simulink model "Khaldoun_Multivariable"  (Simulink 7.9)
settings: Solver=ode45  StartTime=0.0  StopTime=1.5  RelTol=1e-3
InitFcn:
  | k = 1.381e-23;
  | q = 1.602e-19;
  | A = 1.81;
  | Eg = 1.16;
  | Ns = 72;
  | Np=1;
  | ki=1.96e-3;
  | Rs =2.48e-3;
  | Rp = 8.7;
  | Tr =298.5;
  | I0_r = 1.13e-6;
  | Ir_ph = 5.61;
  | 
  | T=298.5;
  | 
  | Ts_Power=5e-6;
  | Ts=5e-6;
  | Ts_Control=10e-6;
  | 
  | Ci=100;
  | C1i=42;
  | D0=0.5;
  | 
  | C=440e-6;
  | L=440e-6;
  | C1=22e-6;
  | 
  | sol=1;
  | 
  | C_init=100;
  | C1_init=42;
  | L1_init=5;
  | 
  | 
  | kg=0.005;
  | a=0.02;
  | wl=50;
  | wh=45;
  | 
  | w1=4500;
  | w2=6500;
  | w3=8500;
  | w4=5500;
  | w5=7500;
  | w6=9500;
StartFcn:
  | k = 1.381e-23;
  | q = 1.602e-19;
  | A = 1.81;
  | Eg = 1.16;
  | Ns = 72;
  | Np=1;
  | ki=1.96e-3;
  | Rs =2.48e-3;
  | Rp = 8.7;
  | Tr =298.5;
  | I0_r = 1.13e-6;
  | Ir_ph = 5.61;
  | 
  | T=298.5;
  | 
  | Ts_Power=5e-6;
  | Ts=5e-6;
  | Ts_Control=10e-6;
  | 
  | Ci=100;
  | C1i=42;
  | D0=0.5;
  | 
  | C=440e-6;
  | L=440e-6;
  | C1=22e-6;
  | 
  | sol=1;
  | 
  | C_init=100;
  | C1_init=42;
  | L1_init=5;
  | 
  | 
  | 
  | kg=0.005;
  | a=0.02;
  | wl=50;
  | wh=45;
  | 
  | w1=4500;
  | w2=6500;
  | w3=8500;
  | w4=5500;
  | w5=7500;
  | w6=9500;
undefined symbols (not defined in the file or in its folder): D1, Delta, sigbuilder_block
libraries: powerlib x99, powerlib_extras x3, simulink x2
(part 1 of 2)
settings Model: Creator=Khaled  LastModifiedBy=Khaled

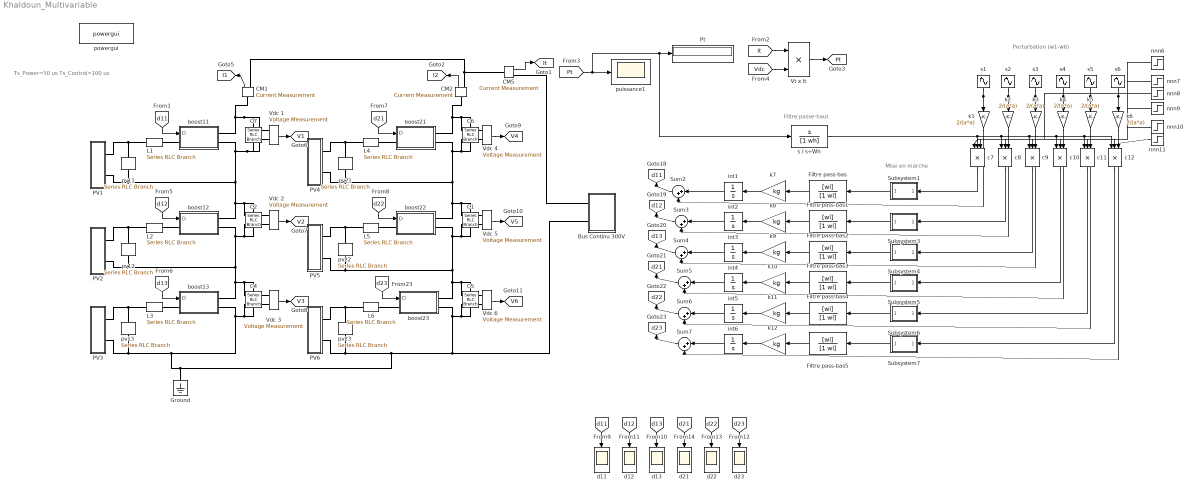
== system Khaldoun_Multivariable ==
  note: Ts_Power=50 us
      | Ts_Control=100 us
  note: Filtre passe-haut
  note: Mise en marche
  note: Perturbation (w1-w6)
  Bus Continu 300V : Subsystem
  C{1..2,4..7} (6 alike) : powerlib/Elements/Series RLC Branch  LConnTagsString=__new0  RConnTagsString=__new0  BranchType=C  Resistance=1.0  Inductance=1.0  SetiL0=off  InitialCurrent=0  Capacitance=C  Setx0=on  InitialVoltage=Ci  Measurements=None
  CM1 : powerlib/Measurements/Current Measurement  Tag=PoWeRsYsTeMmEaSuReMeNt  PhasorSimulation=off  OutputType=Magnitude  PSBequivalent=0
  CM2 : powerlib/Measurements/Current Measurement  Tag=PoWeRsYsTeMmEaSuReMeNt  PhasorSimulation=off  OutputType=Magnitude  PSBequivalent=0
  CM5 : powerlib/Measurements/Current Measurement  Tag=PoWeRsYsTeMmEaSuReMeNt  PhasorSimulation=off  OutputType=Magnitude  PSBequivalent=0
  Filtre pass-bas{,1..5} (6 alike) : TransferFcn  Numerator=[wl]  Denominator=[1 wl]
  Ground : powerlib/Elements/Ground  LConnTagsString=a
  L{1..6} (6 alike) : powerlib/Elements/Series RLC Branch  LConnTagsString=__new0  RConnTagsString=__new0  BranchType=L  Resistance=1.0  Inductance=L  SetiL0=on  InitialCurrent=L1_init  Capacitance=1.0  Setx0=off  InitialVoltage=0  Measurements=None
  PV1 : Subsystem  RequirementInfo={} %GIDa_ec48a4a5_e8ed_46b8_b352_e7f6805c7ac6
  PV2 : Subsystem  RequirementInfo={} %GIDa_9735ab26_5599_4b61_891e_3252a34807da
  PV3 : Subsystem  RequirementInfo={} %GIDa_8edbe910_4089_49ae_850f_62c7b8a72111
  PV4 : Subsystem  RequirementInfo={} %GIDa_f6f8a1f9_a3e9_414c_b28d_369a8e09ef45
  PV5 : Subsystem  RequirementInfo={} %GIDa_1a594654_d930_4a6d_9a1b_d857bde8c8a5
  PV6 : Subsystem  RequirementInfo={} %GIDa_cee78ba7_daff_4548_90a5_e4e442d265c0
  Pt : Display
      settings: Format=bank  Decimation=100
  Subsystem1 : Subsystem
  Subsystem3 : Subsystem
  Subsystem4 : Subsystem
  Subsystem5 : Subsystem
  Subsystem6 : Subsystem
  Subsystem7 : Subsystem
  Sum{2..7} (6 alike) : Sum  Inputs=|++
  Vdc {1..6} (6 alike) : powerlib/Measurements/Voltage Measurement  Tag=PoWeRsYsTeMmEaSuReMeNt  PhasorSimulation=off  OutputType=Magnitude  PSBequivalent=0
  Vt x It : Product  RndMeth=Zero
  boost11 : Subsystem
  boost12 : Subsystem
  boost13 : Subsystem
  boost21 : Subsystem
  boost22 : Subsystem
  boost23 : Subsystem
  c{7..12} (6 alike) : Product  Inputs=3  RndMeth=Zero
  d{11..13,21..23} (6 alike) : Scope
      d11 settings: TimeRange=1  YMin=582  YMax=599  SaveName=mv6  Decimation=100
      d12 settings: TimeRange=1  YMin=582  YMax=599  SaveName=mv1  Decimation=100
      d13 settings: TimeRange=1  YMin=582  YMax=599  SaveName=mv2  Decimation=100
      d21 settings: TimeRange=1  YMin=582  YMax=599  SaveName=mv3  Decimation=100
      d22 settings: TimeRange=1  YMin=582  YMax=599  SaveName=mv4  Decimation=100
      d23 settings: TimeRange=1  YMin=582  YMax=599  SaveName=mv5  Decimation=100
  int{1..6} (6 alike) : Integrator  InitialCondition=0.5  LimitOutput=on  UpperSaturationLimit=0.8  LowerSaturationLimit=0.2
  k{1..6} (6 alike) : Gain  Gain=2/(a*a)
  k{7..12} (6 alike) : Gain  Gain=kg
  nnn{6..11} (6 alike) : Step  Time=0.2  SampleTime=0
  powergui : powerlib/powergui  Priority=1  SimulationMode=Discrete  SolverType=Tustin  SampleTime=Ts_Power  frequency=60  SPID=off  DisableSnubberDevices=off  DisableRonSwitches=off  DisableVfSwitches=off  SwTol=0  Interpol=off  DisplayEquations=off  FunctionMessages=off  frequencyindice=0  Pbase=100e6  ErrMax=1e-4  Iterations=50  UnitsV=kV  UnitsW=MW  echomessages=off  HookPort=off  EnableUseOfTLC=off  x0status=blocks  RestoreLinks=warning  ResistiveCurrentMeasurement=off  Frange=[0:2:500]  Ylog=off  Xlog=on  ShowGrid=off  save=off  variable=ZData  ZoomFFT=on  StartTime=0.0  cycles=1  DisplayStyle=1  fundamental=60  FreqAxis=off  MaxFrequency=1000  frequencyindicesteady=1  RmsSteady=1  display=off  Ts=0  methode=off
  puissance1 : Scope
      settings: TimeRange=1  YMin=0  YMax=1400  SaveName=mv  Decimation=100
  pv{11..13,21..23} (6 alike) : powerlib/Elements/Series RLC Branch  LConnTagsString=__new0  RConnTagsString=__new0  BranchType=C  Resistance=0.01  Inductance=1.0  SetiL0=off  InitialCurrent=0  Capacitance=C1  Setx0=on  InitialVoltage=C1_init  Measurements=None
  s / s+Wh : TransferFcn  Numerator=[1 0]  Denominator=[1 wh]  AbsoluteTolerance=1e-6
  s1 : Sin  Amplitude=a  Frequency=w1/(2*pi)  SampleTime=0
  s2 : Sin  Amplitude=a  Frequency=w2/(2*pi)  SampleTime=0
  s3 : Sin  Amplitude=a  Frequency=w3/(2*pi)  SampleTime=0
  s4 : Sin  Amplitude=a  Frequency=w4/(2*pi)  SampleTime=0
  s5 : Sin  Amplitude=a  Frequency=w5/(2*pi)  SampleTime=0
  s6 : Sin  Amplitude=a  Frequency=w6/(2*pi)  SampleTime=0
  tag scope: I1=global, I2=global, It=global, Pt=global, V1=global, V2=global, V3=global, V4=global, V5=global, V6=global, d11=global, d12=global, d13=global, d21=global, d22=global, d23=global
  wires:
  [It] -> Vt x It/1
  Vt x It/1 -> [Pt]
  [Vdc] -> Vt x It/2
  [Pt] -> puissance1/1, Pt/1, s / s+Wh/1
  s1/1 -> k1/1, Sum2/2
  s2/1 -> k2/1, Sum3/2
  s3/1 -> k3/1, Sum4/2
  s4/1 -> k4/1, Sum5/2
  s5/1 -> k5/1, Sum6/2
  s6/1 -> k6/1, Sum7/2
  k1/1 -> c7/2
  k2/1 -> c8/2
  k3/1 -> c9/2
  k4/1 -> c10/2
  k5/1 -> c11/2
  k6/1 -> c12/2
  c7/1 -> Subsystem1/1(In1)
  c8/1 -> Subsystem3/1(In1)
  c9/1 -> Subsystem4/1(In1)
  c10/1 -> Subsystem5/1(In1)
  c11/1 -> Subsystem6/1(In1)
  c12/1 -> Subsystem7/1(In1)
  Filtre pass-bas/1 -> k7/1
  Filtre pass-bas1/1 -> k8/1
  Filtre pass-bas2/1 -> k9/1
  Filtre pass-bas3/1 -> k10/1
  Filtre pass-bas4/1 -> k11/1
  Filtre pass-bas5/1 -> k12/1
  k7/1 -> int1/1
  k8/1 -> int2/1
  k9/1 -> int3/1
  k10/1 -> int4/1
  k11/1 -> int5/1
  k12/1 -> int6/1
  int1/1 -> Sum2/1
  int2/1 -> Sum3/1
  int3/1 -> Sum4/1
  int4/1 -> Sum5/1
  int5/1 -> Sum6/1
  int6/1 -> Sum7/1
  Sum2/1 -> [d11]
  Sum3/1 -> [d12]
  Sum4/1 -> [d13]
  Sum5/1 -> [d21]
  Sum6/1 -> [d22]
  Sum7/1 -> [d23]
  nnn6/1 -> c7/3
  nnn7/1 -> c8/3
  nnn8/1 -> c9/3
  nnn9/1 -> c10/3
  nnn10/1 -> c11/3
  nnn11/1 -> c12/3
  Subsystem1/1(Out1) -> Filtre pass-bas/1
  Subsystem3/1(Out1) -> Filtre pass-bas1/1
  Subsystem4/1(Out1) -> Filtre pass-bas2/1
  Subsystem5/1(Out1) -> Filtre pass-bas3/1
  Subsystem6/1(Out1) -> Filtre pass-bas4/1
  Subsystem7/1(Out1) -> Filtre pass-bas5/1
  s / s+Wh/1 -> c7/1, c8/1, c9/1, c10/1, c11/1, c12/1
  CM5/1 -> [It]
  CM1/1 -> [I1]
  CM2/1 -> [I2]
  Vdc 1/1 -> [V1]
  Vdc 2/1 -> [V2]
  Vdc 3/1 -> [V3]
  Vdc 6/1 -> [V6]
  Vdc 5/1 -> [V5]
  Vdc 4/1 -> [V4]
  [d11] -> d11/1
  [d12] -> d12/1
  [d13] -> d13/1
  [d21] -> d21/1
  [d22] -> d22/1
  [d23] -> d23/1
  [d11] -> boost11/1(D)
  [d12] -> boost12/1(D)
  [d13] -> boost13/1(D)
  [d21] -> boost21/1(D)
  [d22] -> boost22/1(D)
  [d23] -> boost23/1(D)
  connections:
  PV2/RConn1 -- pv12/LConn1 -- L2/RConn1
  PV3/RConn1 -- L3/RConn1 -- pv13/LConn1
  pv11/RConn1 -- PV1/RConn2 -- boost11/RConn2 -- Vdc 1/LConn2 -- C7/RConn1 -- boost12/RConn1 -- Vdc 2/LConn1 -- C2/LConn1
  boost13/RConn1 -- pv12/RConn1 -- PV2/RConn2 -- Vdc 2/LConn2 -- C2/RConn1 -- boost12/RConn2 -- Vdc 3/LConn1 -- C4/LConn1
  PV1/RConn1 -- L1/RConn1 -- pv11/LConn1
  PV5/RConn1 -- pv22/LConn1 -- L5/RConn1
  PV6/RConn1 -- L6/RConn1 -- pv23/LConn1
  boost22/RConn1 -- C6/RConn1 -- Vdc 4/LConn2 -- boost21/RConn2 -- pv21/RConn1 -- PV4/RConn2 -- Vdc 5/LConn1 -- C1/LConn1
  C6/LConn1 -- Vdc 4/LConn1 -- CM2/LConn1 -- boost21/RConn1
  boost23/RConn1 -- pv22/RConn1 -- PV5/RConn2 -- Vdc 5/LConn2 -- C1/RConn1 -- boost22/RConn2 -- Vdc 6/LConn1 -- C5/LConn1
  PV4/RConn1 -- L4/RConn1 -- pv21/LConn1
  CM1/LConn1 -- boost11/RConn1 -- Vdc 1/LConn1 -- C7/LConn1
  CM5/LConn1 -- CM2/RConn1 -- CM1/RConn1
  boost13/RConn2 -- pv13/RConn1 -- PV3/RConn2 -- pv23/RConn1 -- PV6/RConn2 -- Vdc 6/LConn2 -- C5/RConn1 -- boost23/RConn2 -- Bus Continu 300V/LConn2 -- Ground/LConn1 -- Vdc 3/LConn2 -- C4/RConn1
  L3/LConn1 -- boost13/LConn1
  Bus Continu 300V/LConn1 -- CM5/RConn1
  boost21/LConn1 -- L4/LConn1
  L2/LConn1 -- boost12/LConn1
  boost11/LConn1 -- L1/LConn1
  L6/LConn1 -- boost23/LConn1
  L5/LConn1 -- boost22/LConn1

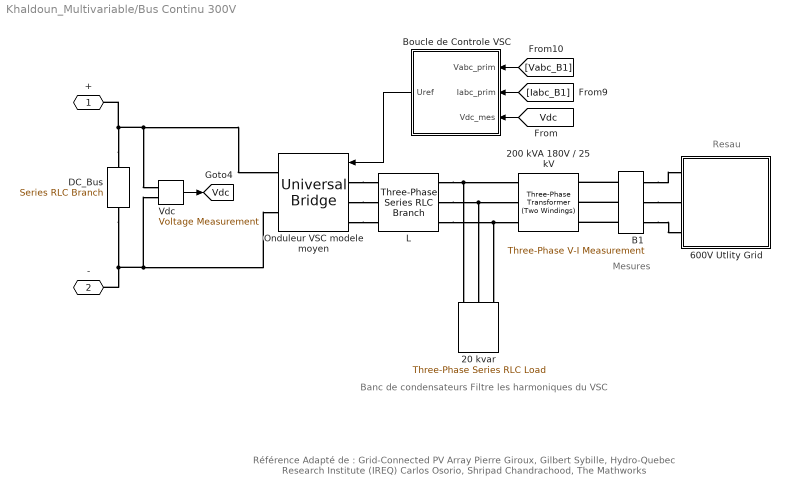
== system Khaldoun_Multivariable/Bus Continu 300V ==
  note: Resau
  note: Banc de condensateurs
      | Filtre les harmoniques du VSC
  note: Mesures
  note: Référence
      | Adapté de :
      | Grid-Connected PV Array
      | Pierre Giroux, Gilbert Sybille, Hydro-Quebec Research Institute (IREQ) Carlos Osorio, Shripad Chandrachood, The Mathworks
  "20 kvar " : powerlib/Elements/Three-Phase Series RLC Load  LConnTagsString=A|B|C  Configuration=Y (grounded)  NominalVoltage=180  NominalFrequency=60  ActivePower=20e3/100  InductivePower=0  CapacitivePower=20e3  Measurements=None  LoadType=constant Z
  200 kVA 180V / 25 kV : powerlib/Elements/Three-Phase Transformer (Two Windings)  Winding1Connection=Yg  UNITS=pu  NominalPower=[200e3 , 60 ]  Winding1=[ 25e3 , 0.001 , 0.03 ]  Winding2Connection=Delta (D1)  Winding2=[ 180 , 0.001 , 0.03 ]  SetSaturation=off  Rm=500  Lm=500  Saturation=[ 0,0 ; 0.0024,1.2 ; 1.0,1.52 ]  Hysteresis=off  DataFile='hysteresis'  SetInitialFlux=off  InitialFluxes=[ 0.8 , -0.8 , 0.7 ]  Measurements=None  MoreParameters=off  BreakLoop=off  DataType=off  TransfoNumber=0
  600V Utlity Grid : Subsystem
  B1 : powerlib/Measurements/Three-Phase V-I Measurement  VoltageMeasurement=phase-to-ground  SetLabelV=on  LabelV=Vabc_B1  Vpu=off  VpuLL=off  CurrentMeasurement=yes  SetLabelI=on  LabelI=Iabc_B1  Ipu=off  Pbase=100e6  Vbase=500e3  OutputType=Magnitude  PhasorSimulation=off  PSBequivalent=0
  Boucle de Controle VSC : Subsystem  mask(VSC Main Controller){nom=[ 200e3  60 ], Vnom=[ 25e3 260 ], Vnom_dc=300, RLxfo=[0.002  0.06 ], RLchoke=[1e-3  125e-6  ], K_VDCreg=[2  800], K_Ireg=[0.3 20], Ts=Ts_Control}
      mask prompts: nom "Puissance et féquence nominales [ Pnom(VA)  Fnom(Hz) ]:"; Vnom "Tension nominale au primaire et secondaire (Vrms LL) [ Vnom_prim   Vnom_sec ]:"; Vnom_dc "Tension du bus DC bus nominale (V):"; RLxfo "Impedance de fuite du transformateur (pu/Pnom) [ Rxfo  Lxf ]"; RLchoke "Impedance choke [ R(ohm) L(H) ]"; K_VDCreg "Gains régulateur de tension du bus DC [ Kp  Ki ]:"; K_Ireg "Gains régulateur du courant du bus D [ Kp  Ki ]:"; Ts "Temps d'échantillonnage"
      mask init:
      | Pnom=nom(1);
      | Fnom=nom(2);
      | Vnom_prim=Vnom(1);
      | Vnom_sec=Vnom(2);
      | Zbase=Vnom_sec^2/Pnom;
      | Rtot_pu=RLxfo(1) + RLchoke(1)/Zbase;
      | Ltot_pu=RLxfo(2) + RLchoke(2)/(Zbase/(2*pi*Fnom));
      | Kp_VDCreg=K_VDCreg(1);
      | Ki_VDCreg=K_VDCreg(2);
      | Kp_Ireg=K_Ireg(1);
      | Ki_Ireg=K_Ireg(2);
      | Vdc_ref=Vnom_dc;
  DC_Bus : powerlib/Elements/Series RLC Branch  LConnTagsString=__new0  RConnTagsString=__new0  BranchType=C  Resistance=1.0  Inductance=1.0  SetiL0=off  InitialCurrent=0  Capacitance=12000e-6  Setx0=on  InitialVoltage=300  Measurements=None
  L : powerlib/Elements/Three-Phase Series RLC Branch  LConnTagsString=A|B|C  RConnTagsString=A|B|C  BranchType=RL  Resistance=0.1  Inductance=125e-6  Capacitance=inf  Measurements=None
  Onduleur VSC modele moyen : powerlib/Power Electronics/Universal Bridge  Arms=3  SnubberResistance=1e5  SnubberCapacitance=inf  Device=Average-model based VSC  Ron=1e-3  Lon=0  ForwardVoltages="[  0  0  ]"  ForwardVoltage=0  GTOparameters=[ 10e-6 , 20e-6 ]  IGBTparameters=[ 1e-6 , 2e-6 ]  Measurements=None  Measurements_2=None  converterType=Rectifier
  "Vdc " : powerlib/Measurements/Voltage Measurement  Tag=PoWeRsYsTeMmEaSuReMeNt  PhasorSimulation=off  OutputType=Magnitude  PSBequivalent=0
  + : PMIOPort  Port=1  Side=Left
  - : PMIOPort  Port=2  Side=Left
  tag scope: Vdc=global
  wires:
  [Vabc_B1] -> Boucle de Controle VSC/1(Vabc_prim)
  [Iabc_B1] -> Boucle de Controle VSC/2(Iabc_prim)
  [Vdc] -> Boucle de Controle VSC/3(Vdc_mes)
  Boucle de Controle VSC/1(Uref) -> Onduleur VSC modele moyen/1
  "Vdc "/1 -> [Vdc]
  connections:
  L/RConn1 -- "20 kvar "/LConn1 -- 200 kVA 180V / 25 kV/RConn1
  L/RConn2 -- "20 kvar "/LConn2 -- 200 kVA 180V / 25 kV/RConn2
  L/RConn3 -- "20 kvar "/LConn3 -- 200 kVA 180V / 25 kV/RConn3
  B1/LConn1 -- 200 kVA 180V / 25 kV/LConn1
  B1/LConn2 -- 200 kVA 180V / 25 kV/LConn2
  B1/LConn3 -- 200 kVA 180V / 25 kV/LConn3
  B1/RConn1 -- 600V Utlity Grid/LConn1
  B1/RConn2 -- 600V Utlity Grid/LConn2
  B1/RConn3 -- 600V Utlity Grid/LConn3
  DC_Bus/LConn1 -- +/RConn1 -- Onduleur VSC modele moyen/RConn1 -- "Vdc "/LConn1
  DC_Bus/RConn1 -- -/RConn1 -- Onduleur VSC modele moyen/RConn2 -- "Vdc "/LConn2
  Onduleur VSC modele moyen/LConn1 -- L/LConn1
  Onduleur VSC modele moyen/LConn2 -- L/LConn2
  Onduleur VSC modele moyen/LConn3 -- L/LConn3

== system Khaldoun_Multivariable/PV1 ==
  Diode : Subsystem
      mask Display:
      | plot(-75,-50,100,150, [-15 -15 43 -15 -15 -75],[50 8 50 92 50 50], ...
      |     [43 43],[8 94],[100 43], [50 50])
  Eclairage : Step  Time=0  Before=1  SampleTime=0
  Iph : powerlib/Electrical Sources/Controlled Current Source  Initialize=on  Source_Type=DC  Amplitude=0  Phase=0  Frequency=0  Measurements=None
  Iph_ : Constant  Value=Ir_ph
  Product1 : Product  Inputs=**  RndMeth=Zero
  Rp : powerlib/Elements/Series RLC Branch  LConnTagsString=__new0  RConnTagsString=__new0  BranchType=R  Resistance=8.7*72  Inductance=1e-3  SetiL0=off  InitialCurrent=0  Capacitance=1e-6  Setx0=off  InitialVoltage=0  Measurements=Branch current
  Rs : powerlib/Elements/Series RLC Branch  LConnTagsString=__new0  RConnTagsString=__new0  BranchType=R  Resistance=2.48e-3  Inductance=1e-3  SetiL0=off  InitialCurrent=0  Capacitance=1e-6  Setx0=off  InitialVoltage=0  Measurements=None
  x1000 : Gain
  + : PMIOPort  Port=1  Side=Right
  - : PMIOPort  Port=2  Side=Right
  wires:
  Eclairage/1 -> x1000/1
  Product1/1 -> Iph/1
  Iph_/1 -> Product1/1
  x1000/1 -> Product1/2
  connections:
  Iph/RConn1 -- Diode/LConn1 -- Rs/LConn1 -- Rp/LConn1
  Rp/RConn1 -- -/RConn1 -- Iph/LConn1 -- Diode/RConn1
  +/RConn1 -- Rs/RConn1

== system Khaldoun_Multivariable/PV2 ==
  Diode : Subsystem
      mask Display:
      | plot(-75,-50,100,150, [-15 -15 43 -15 -15 -75],[50 8 50 92 50 50], ...
      |     [43 43],[8 94],[100 43], [50 50])
  Eclairage (W/m2) : Subsystem  Tag=STV Subsys  LoadFcn=sigbuilder_block('load');  StartFcn=sigbuilder_block('start');  StopFcn=sigbuilder_block('stop');  ClipboardFcn=sigbuilder_block('clipboard');  mask(Sigbuilder block){}
      mask help: Sigbuilder GUI
      mask init:
      | if ~strcmp(get_param(bdroot(gcbh),'SimulationStatus'),'stopped') tuvar = sigbuilder_block('maskInit'); end
      settings: CopyFcn=sigbuilder_block('copy');  DeleteFcn=sigbuilder_block('delete');  ModelCloseFcn=sigbuilder_block('modelClose');  PreSaveFcn=sigbuilder_block('preSave');  PauseFcn=sigbuilder_block('pause')  ContinueFcn=sigbuilder_block('continue')  NameChangeFcn=sigbuilder_block('namechange');  OpenFcn=sigbuilder_block('open',[35.25 78 954 513.75 ]);  CloseFcn=sigbuilder_block('close');
      mask Display: plot(0,0,100,100,[10,10,40,40,10],[80,20,20,80,80],[40,10],[50,50], [40,27,10],[65,72,56],[40,25,25,10],[28,28,43,43]);
  Iph : powerlib/Electrical Sources/Controlled Current Source  Initialize=on  Source_Type=DC  Amplitude=0  Phase=0  Frequency=0  Measurements=None
  Iph_ : Constant  Value=Ir_ph
  Product1 : Product  Inputs=**  RndMeth=Zero
  Rp : powerlib/Elements/Series RLC Branch  LConnTagsString=__new0  RConnTagsString=__new0  BranchType=R  Resistance=8.7*72  Inductance=1e-3  SetiL0=off  InitialCurrent=0  Capacitance=1e-6  Setx0=off  InitialVoltage=0  Measurements=Branch current
  Rs : powerlib/Elements/Series RLC Branch  LConnTagsString=__new0  RConnTagsString=__new0  BranchType=R  Resistance=2.48e-3  Inductance=1e-3  SetiL0=off  InitialCurrent=0  Capacitance=1e-6  Setx0=off  InitialVoltage=0  Measurements=None
  x1000 : Gain
  + : PMIOPort  Port=1  Side=Right
  - : PMIOPort  Port=2  Side=Right
  wires:
  Eclairage (W/m2)/1(Ir) -> x1000/1
  Product1/1 -> Iph/1
  Iph_/1 -> Product1/1
  x1000/1 -> Product1/2
  connections:
  Iph/RConn1 -- Diode/LConn1 -- Rs/LConn1 -- Rp/LConn1
  Rp/RConn1 -- -/RConn1 -- Iph/LConn1 -- Diode/RConn1
  +/RConn1 -- Rs/RConn1

== system Khaldoun_Multivariable/PV3 ==
  Diode : Subsystem
      mask Display:
      | plot(-75,-50,100,150, [-15 -15 43 -15 -15 -75],[50 8 50 92 50 50], ...
      |     [43 43],[8 94],[100 43], [50 50])
  Eclairage : Step  Time=0  Before=1  SampleTime=0
  Iph : powerlib/Electrical Sources/Controlled Current Source  Initialize=on  Source_Type=DC  Amplitude=0  Phase=0  Frequency=0  Measurements=None
  Iph_ : Constant  Value=Ir_ph
  Product1 : Product  Inputs=**  RndMeth=Zero
  Rp : powerlib/Elements/Series RLC Branch  LConnTagsString=__new0  RConnTagsString=__new0  BranchType=R  Resistance=8.7*72  Inductance=1e-3  SetiL0=off  InitialCurrent=0  Capacitance=1e-6  Setx0=off  InitialVoltage=0  Measurements=Branch current
  Rs : powerlib/Elements/Series RLC Branch  LConnTagsString=__new0  RConnTagsString=__new0  BranchType=R  Resistance=2.48e-3  Inductance=1e-3  SetiL0=off  InitialCurrent=0  Capacitance=1e-6  Setx0=off  InitialVoltage=0  Measurements=None
  x1000 : Gain
  + : PMIOPort  Port=1  Side=Right
  - : PMIOPort  Port=2  Side=Right
  wires:
  x1000/1 -> Product1/2
  Iph_/1 -> Product1/1
  Product1/1 -> Iph/1
  Eclairage/1 -> x1000/1
  connections:
  +/RConn1 -- Rs/RConn1
  Diode/RConn1 -- Iph/LConn1 -- -/RConn1 -- Rp/RConn1
  Rp/LConn1 -- Rs/LConn1 -- Diode/LConn1 -- Iph/RConn1

== system Khaldoun_Multivariable/PV4 ==
  Diode : Subsystem
      mask Display:
      | plot(-75,-50,100,150, [-15 -15 43 -15 -15 -75],[50 8 50 92 50 50], ...
      |     [43 43],[8 94],[100 43], [50 50])
  Eclairage : Step  Time=0  Before=1  SampleTime=0
  Iph : powerlib/Electrical Sources/Controlled Current Source  Initialize=on  Source_Type=DC  Amplitude=0  Phase=0  Frequency=0  Measurements=None
  Iph_ : Constant  Value=Ir_ph
  Product1 : Product  Inputs=**  RndMeth=Zero
  Rp : powerlib/Elements/Series RLC Branch  LConnTagsString=__new0  RConnTagsString=__new0  BranchType=R  Resistance=8.7*72  Inductance=1e-3  SetiL0=off  InitialCurrent=0  Capacitance=1e-6  Setx0=off  InitialVoltage=0  Measurements=Branch current
  Rs : powerlib/Elements/Series RLC Branch  LConnTagsString=__new0  RConnTagsString=__new0  BranchType=R  Resistance=2.48e-3  Inductance=1e-3  SetiL0=off  InitialCurrent=0  Capacitance=1e-6  Setx0=off  InitialVoltage=0  Measurements=None
  x1000 : Gain
  + : PMIOPort  Port=1  Side=Right
  - : PMIOPort  Port=2  Side=Right
  wires:
  Eclairage/1 -> x1000/1
  Product1/1 -> Iph/1
  Iph_/1 -> Product1/1
  x1000/1 -> Product1/2
  connections:
  Iph/RConn1 -- Diode/LConn1 -- Rs/LConn1 -- Rp/LConn1
  Rp/RConn1 -- -/RConn1 -- Iph/LConn1 -- Diode/RConn1
  +/RConn1 -- Rs/RConn1

== system Khaldoun_Multivariable/PV5 ==
  Diode : Subsystem
      mask Display:
      | plot(-75,-50,100,150, [-15 -15 43 -15 -15 -75],[50 8 50 92 50 50], ...
      |     [43 43],[8 94],[100 43], [50 50])
  Eclairage : Step  Time=0  Before=1  SampleTime=0
  Iph : powerlib/Electrical Sources/Controlled Current Source  Initialize=on  Source_Type=DC  Amplitude=0  Phase=0  Frequency=0  Measurements=None
  Iph_ : Constant  Value=Ir_ph
  Product1 : Product  Inputs=**  RndMeth=Zero
  Rp : powerlib/Elements/Series RLC Branch  LConnTagsString=__new0  RConnTagsString=__new0  BranchType=R  Resistance=8.7*72  Inductance=1e-3  SetiL0=off  InitialCurrent=0  Capacitance=1e-6  Setx0=off  InitialVoltage=0  Measurements=Branch current
  Rs : powerlib/Elements/Series RLC Branch  LConnTagsString=__new0  RConnTagsString=__new0  BranchType=R  Resistance=2.48e-3  Inductance=1e-3  SetiL0=off  InitialCurrent=0  Capacitance=1e-6  Setx0=off  InitialVoltage=0  Measurements=None
  x1000 : Gain
  + : PMIOPort  Port=1  Side=Right
  - : PMIOPort  Port=2  Side=Right
  wires:
  x1000/1 -> Product1/2
  Iph_/1 -> Product1/1
  Product1/1 -> Iph/1
  Eclairage/1 -> x1000/1
  connections:
  +/RConn1 -- Rs/RConn1
  Diode/RConn1 -- Iph/LConn1 -- -/RConn1 -- Rp/RConn1
  Rp/LConn1 -- Rs/LConn1 -- Diode/LConn1 -- Iph/RConn1

== system Khaldoun_Multivariable/PV6 ==
  Diode : Subsystem
      mask Display:
      | plot(-75,-50,100,150, [-15 -15 43 -15 -15 -75],[50 8 50 92 50 50], ...
      |     [43 43],[8 94],[100 43], [50 50])
  Eclairage (W/m2) : Subsystem  Tag=STV Subsys  LoadFcn=sigbuilder_block('load');  StartFcn=sigbuilder_block('start');  StopFcn=sigbuilder_block('stop');  ClipboardFcn=sigbuilder_block('clipboard');  mask(Sigbuilder block){}
      mask help: Sigbuilder GUI
      mask init:
      | if ~strcmp(get_param(bdroot(gcbh),'SimulationStatus'),'stopped') tuvar = sigbuilder_block('maskInit'); end
      settings: CopyFcn=sigbuilder_block('copy');  DeleteFcn=sigbuilder_block('delete');  ModelCloseFcn=sigbuilder_block('modelClose');  PreSaveFcn=sigbuilder_block('preSave');  PauseFcn=sigbuilder_block('pause')  ContinueFcn=sigbuilder_block('continue')  NameChangeFcn=sigbuilder_block('namechange');  OpenFcn=sigbuilder_block('open',[35.25 78 954 513.75 ]);  CloseFcn=sigbuilder_block('close');
      mask Display: plot(0,0,100,100,[10,10,40,40,10],[80,20,20,80,80],[40,10],[50,50], [40,27,10],[65,72,56],[40,25,25,10],[28,28,43,43]);
  Iph : powerlib/Electrical Sources/Controlled Current Source  Initialize=on  Source_Type=DC  Amplitude=0  Phase=0  Frequency=0  Measurements=None
  Iph_ : Constant  Value=Ir_ph
  Product1 : Product  Inputs=**  RndMeth=Zero
  Rp : powerlib/Elements/Series RLC Branch  LConnTagsString=__new0  RConnTagsString=__new0  BranchType=R  Resistance=8.7*72  Inductance=1e-3  SetiL0=off  InitialCurrent=0  Capacitance=1e-6  Setx0=off  InitialVoltage=0  Measurements=Branch current
  Rs : powerlib/Elements/Series RLC Branch  LConnTagsString=__new0  RConnTagsString=__new0  BranchType=R  Resistance=2.48e-3  Inductance=1e-3  SetiL0=off  InitialCurrent=0  Capacitance=1e-6  Setx0=off  InitialVoltage=0  Measurements=None
  x1000 : Gain
  + : PMIOPort  Port=1  Side=Right
  - : PMIOPort  Port=2  Side=Right
  wires:
  x1000/1 -> Product1/2
  Iph_/1 -> Product1/1
  Product1/1 -> Iph/1
  Eclairage (W/m2)/1(Ir) -> x1000/1
  connections:
  +/RConn1 -- Rs/RConn1
  Diode/RConn1 -- Iph/LConn1 -- -/RConn1 -- Rp/RConn1
  Rp/LConn1 -- Rs/LConn1 -- Diode/LConn1 -- Iph/RConn1

== system Khaldoun_Multivariable/Subsystem1 ==
  In1 : Inport
  Add : Sum
  n : Step  Time=0.2  Before=0.5  After=0  SampleTime=0
  nn : Product  RndMeth=Zero
  nnn : Step  Time=0.2  SampleTime=0
  Out1 : Outport
  wires:
  nn/1 -> Add/1
  n/1 -> Add/2
  nnn/1 -> nn/2
  In1/1 -> nn/1
  Add/1 -> Out1/1

== system Khaldoun_Multivariable/Subsystem3 ==
  In1 : Inport
  Add : Sum
  n : Step  Time=0.2  Before=0.5  After=0  SampleTime=0
  nn : Product  RndMeth=Zero
  nnn : Step  Time=0.2  SampleTime=0
  Out1 : Outport
  wires:
  Add/1 -> Out1/1
  In1/1 -> nn/1
  nnn/1 -> nn/2
  n/1 -> Add/2
  nn/1 -> Add/1

== system Khaldoun_Multivariable/Subsystem4 ==
  In1 : Inport
  Add : Sum
  n : Step  Time=0.2  Before=0.5  After=0  SampleTime=0
  nn : Product  RndMeth=Zero
  nnn : Step  Time=0.2  SampleTime=0
  Out1 : Outport
  wires:
  nn/1 -> Add/1
  n/1 -> Add/2
  nnn/1 -> nn/2
  In1/1 -> nn/1
  Add/1 -> Out1/1

== system Khaldoun_Multivariable/Subsystem5 ==
  In1 : Inport
  Add : Sum
  n : Step  Time=0.2  Before=0.5  After=0  SampleTime=0
  nn : Product  RndMeth=Zero
  nnn : Step  Time=0.2  SampleTime=0
  Out1 : Outport
  wires:
  Add/1 -> Out1/1
  In1/1 -> nn/1
  nnn/1 -> nn/2
  n/1 -> Add/2
  nn/1 -> Add/1

== system Khaldoun_Multivariable/Subsystem6 ==
  In1 : Inport
  Add : Sum
  n : Step  Time=0.2  Before=0.5  After=0  SampleTime=0
  nn : Product  RndMeth=Zero
  nnn : Step  Time=0.2  SampleTime=0
  Out1 : Outport
  wires:
  nn/1 -> Add/1
  n/1 -> Add/2
  nnn/1 -> nn/2
  In1/1 -> nn/1
  Add/1 -> Out1/1

== system Khaldoun_Multivariable/Subsystem7 ==
  In1 : Inport
  Add : Sum
  n : Step  Time=0.2  Before=0.5  After=0  SampleTime=0
  nn : Product  RndMeth=Zero
  nnn : Step  Time=0.2  SampleTime=0
  Out1 : Outport
  wires:
  Add/1 -> Out1/1
  In1/1 -> nn/1
  nnn/1 -> nn/2
  n/1 -> Add/2
  nn/1 -> Add/1

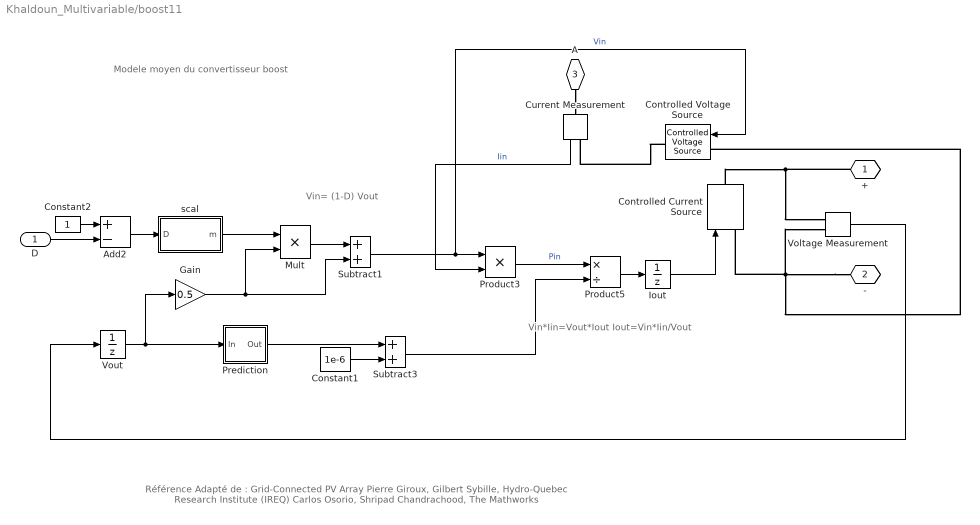
== system Khaldoun_Multivariable/boost11 ==
  note: Vin*Iin=Vout*Iout
      | Iout=Vin*Iin/Vout
  note: Vin= (1-D) Vout
  note: Modele moyen du convertisseur boost
  note: Référence
      | Adapté de :
      | Grid-Connected PV Array
      | Pierre Giroux, Gilbert Sybille, Hydro-Quebec Research Institute (IREQ) Carlos Osorio, Shripad Chandrachood, The Mathworks
  D : Inport
  Add2 : Sum  Inputs=+-
  Constant1 : Constant  Value=1e-6
  Constant2 : Constant
  Controlled Current Source : powerlib/Electrical Sources/Controlled Current Source  Initialize=on  Source_Type=AC  Amplitude=0  Phase=0  Frequency=0  Measurements=None
  Controlled Voltage Source : powerlib/Electrical Sources/Controlled Voltage Source  Initialize=on  Source_Type=AC  Amplitude=0  Phase=0  Frequency=0  Measurements=None
  Current Measurement : powerlib/Measurements/Current Measurement  PhasorSimulation=off  OutputType=Complex  PSBequivalent=0
  Gain : Gain  Gain=0.5
  Iout : UnitDelay  SampleTime=Ts
  Mult : Product  Inputs=**
  Prediction : Subsystem
  Product3 : Product  RndMeth=Zero
  Product5 : Product  Inputs=*/  RndMeth=Zero
  Subtract1 : Sum
  Subtract3 : Sum
  Voltage Measurement : powerlib/Measurements/Voltage Measurement  PhasorSimulation=off  OutputType=Complex  PSBequivalent=0
  Vout : UnitDelay  SampleTime=Ts
  scal : Subsystem
  + : PMIOPort  Tag=PMCPort  Port=1  Side=Right
  - : PMIOPort  Tag=PMCPort  Port=2  Side=Right
  A : PMIOPort  Tag=PMCPort  Port=3  Side=Left
  wires:
  Gain/1 -> Mult/2, Subtract1/2
  Product5/1 -> Iout/1
  Constant1/1 -> Subtract3/2
  Subtract3/1 -> Product5/2
  Product3/1 -> Product5/1  "Pin"
  Prediction/1(Out) -> Subtract3/1
  Vout/1 -> Prediction/1(In), Gain/1
  Subtract1/1 -> Product3/1, Controlled Voltage Source/1  "Vin"
  Mult/1 -> Subtract1/1
  Constant2/1 -> Add2/1
  Add2/1 -> scal/1(D)
  scal/1(m) -> Mult/1
  D/1 -> Add2/2
  Voltage Measurement/1 -> Vout/1
  Iout/1 -> Controlled Current Source/1
  Current Measurement/1 -> Product3/2  "Iin"
  connections:
  -/RConn1 -- Voltage Measurement/LConn2 -- Controlled Voltage Source/LConn1 -- Controlled Current Source/LConn1
  +/RConn1 -- Voltage Measurement/LConn1 -- Controlled Current Source/RConn1
  A/RConn1 -- Current Measurement/LConn1
  Controlled Voltage Source/RConn1 -- Current Measurement/RConn1

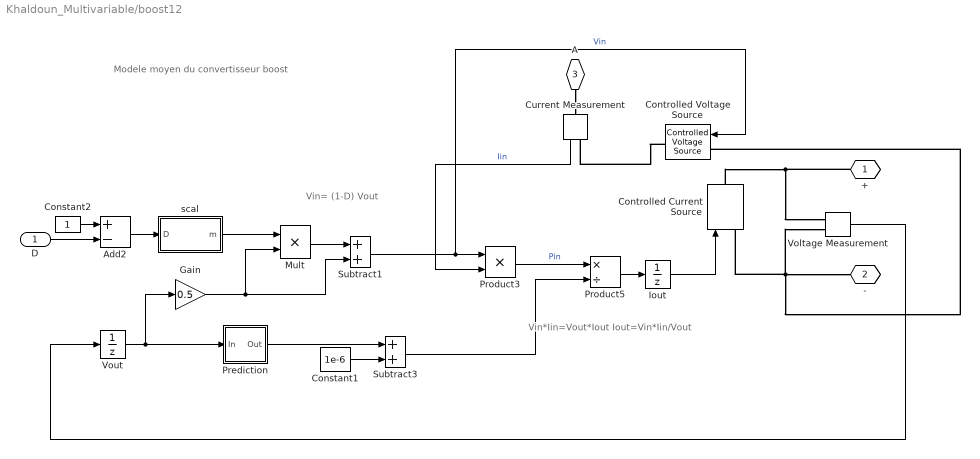
== system Khaldoun_Multivariable/boost12 ==
  note: Modele moyen du convertisseur boost
  note: Vin= (1-D) Vout
  note: Vin*Iin=Vout*Iout
      | Iout=Vin*Iin/Vout
  D : Inport
  Add2 : Sum  Inputs=+-
  Constant1 : Constant  Value=1e-6
  Constant2 : Constant
  Controlled Current Source : powerlib/Electrical Sources/Controlled Current Source  Initialize=on  Source_Type=AC  Amplitude=0  Phase=0  Frequency=0  Measurements=None
  Controlled Voltage Source : powerlib/Electrical Sources/Controlled Voltage Source  Initialize=on  Source_Type=AC  Amplitude=0  Phase=0  Frequency=0  Measurements=None
  Current Measurement : powerlib/Measurements/Current Measurement  PhasorSimulation=off  OutputType=Complex  PSBequivalent=0
  Gain : Gain  Gain=0.5
  Iout : UnitDelay  SampleTime=Ts
  Mult : Product  Inputs=**
  Prediction : Subsystem
  Product3 : Product  RndMeth=Zero
  Product5 : Product  Inputs=*/  RndMeth=Zero
  Subtract1 : Sum
  Subtract3 : Sum
  Voltage Measurement : powerlib/Measurements/Voltage Measurement  PhasorSimulation=off  OutputType=Complex  PSBequivalent=0
  Vout : UnitDelay  SampleTime=Ts
  scal : Subsystem
  + : PMIOPort  Tag=PMCPort  Port=1  Side=Right
  - : PMIOPort  Tag=PMCPort  Port=2  Side=Right
  A : PMIOPort  Tag=PMCPort  Port=3  Side=Left
  wires:
  Current Measurement/1 -> Product3/2  "Iin"
  Iout/1 -> Controlled Current Source/1
  Voltage Measurement/1 -> Vout/1
  D/1 -> Add2/2
  scal/1(m) -> Mult/1
  Add2/1 -> scal/1(D)
  Constant2/1 -> Add2/1
  Mult/1 -> Subtract1/1
  Subtract1/1 -> Controlled Voltage Source/1, Product3/1  "Vin"
  Vout/1 -> Gain/1, Prediction/1(In)
  Prediction/1(Out) -> Subtract3/1
  Product3/1 -> Product5/1  "Pin"
  Subtract3/1 -> Product5/2
  Constant1/1 -> Subtract3/2
  Product5/1 -> Iout/1
  Gain/1 -> Subtract1/2, Mult/2
  connections:
  Controlled Voltage Source/RConn1 -- Current Measurement/RConn1
  A/RConn1 -- Current Measurement/LConn1
  Controlled Current Source/RConn1 -- Voltage Measurement/LConn1 -- +/RConn1
  Controlled Current Source/LConn1 -- Controlled Voltage Source/LConn1 -- Voltage Measurement/LConn2 -- -/RConn1

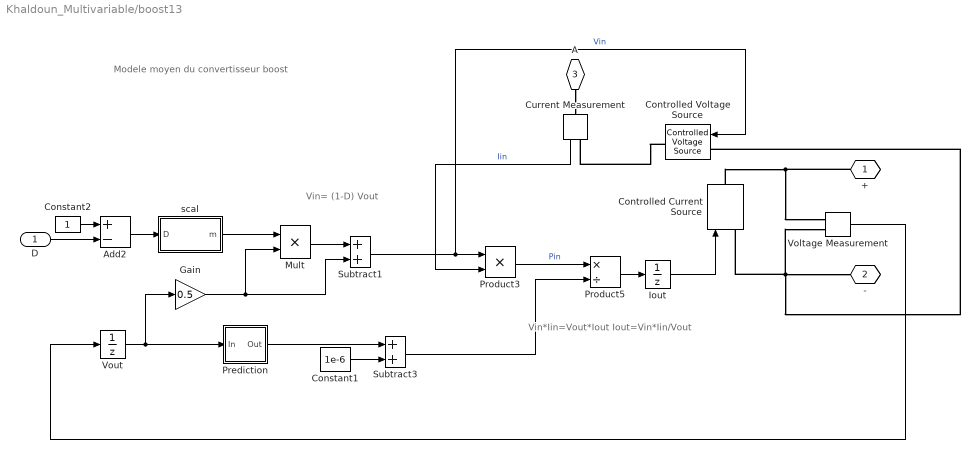
== system Khaldoun_Multivariable/boost13 ==
  note: Modele moyen du convertisseur boost
  note: Vin= (1-D) Vout
  note: Vin*Iin=Vout*Iout
      | Iout=Vin*Iin/Vout
  D : Inport
  Add2 : Sum  Inputs=+-
  Constant1 : Constant  Value=1e-6
  Constant2 : Constant
  Controlled Current Source : powerlib/Electrical Sources/Controlled Current Source  Initialize=on  Source_Type=AC  Amplitude=0  Phase=0  Frequency=0  Measurements=None
  Controlled Voltage Source : powerlib/Electrical Sources/Controlled Voltage Source  Initialize=on  Source_Type=AC  Amplitude=0  Phase=0  Frequency=0  Measurements=None
  Current Measurement : powerlib/Measurements/Current Measurement  PhasorSimulation=off  OutputType=Complex  PSBequivalent=0
  Gain : Gain  Gain=0.5
  Iout : UnitDelay  SampleTime=Ts
  Mult : Product  Inputs=**
  Prediction : Subsystem
  Product3 : Product  RndMeth=Zero
  Product5 : Product  Inputs=*/  RndMeth=Zero
  Subtract1 : Sum
  Subtract3 : Sum
  Voltage Measurement : powerlib/Measurements/Voltage Measurement  PhasorSimulation=off  OutputType=Complex  PSBequivalent=0
  Vout : UnitDelay  SampleTime=Ts
  scal : Subsystem
  + : PMIOPort  Tag=PMCPort  Port=1  Side=Right
  - : PMIOPort  Tag=PMCPort  Port=2  Side=Right
  A : PMIOPort  Tag=PMCPort  Port=3  Side=Left
  wires:
  Current Measurement/1 -> Product3/2  "Iin"
  Iout/1 -> Controlled Current Source/1
  Voltage Measurement/1 -> Vout/1
  D/1 -> Add2/2
  scal/1(m) -> Mult/1
  Add2/1 -> scal/1(D)
  Constant2/1 -> Add2/1
  Mult/1 -> Subtract1/1
  Subtract1/1 -> Controlled Voltage Source/1, Product3/1  "Vin"
  Vout/1 -> Gain/1, Prediction/1(In)
  Prediction/1(Out) -> Subtract3/1
  Product3/1 -> Product5/1  "Pin"
  Subtract3/1 -> Product5/2
  Constant1/1 -> Subtract3/2
  Product5/1 -> Iout/1
  Gain/1 -> Subtract1/2, Mult/2
  connections:
  Controlled Voltage Source/RConn1 -- Current Measurement/RConn1
  A/RConn1 -- Current Measurement/LConn1
  Controlled Current Source/RConn1 -- Voltage Measurement/LConn1 -- +/RConn1
  Controlled Current Source/LConn1 -- Controlled Voltage Source/LConn1 -- Voltage Measurement/LConn2 -- -/RConn1

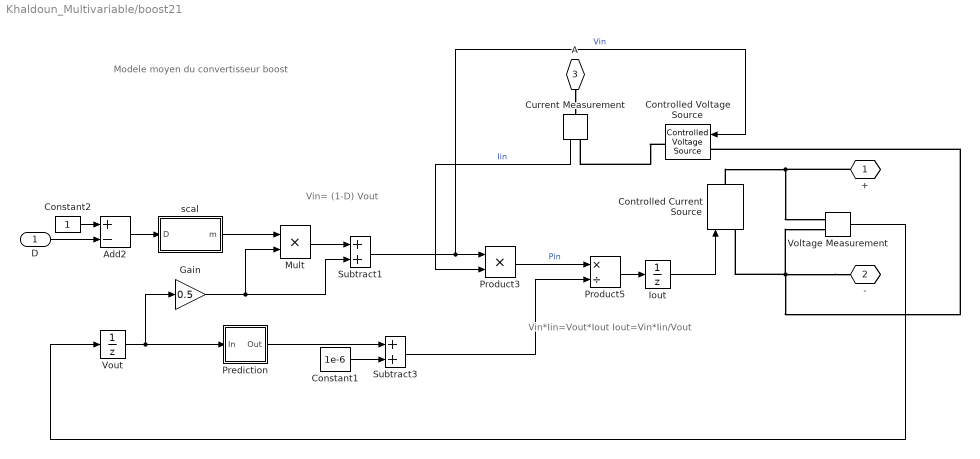
== system Khaldoun_Multivariable/boost21 ==
  note: Vin*Iin=Vout*Iout
      | Iout=Vin*Iin/Vout
  note: Vin= (1-D) Vout
  note: Modele moyen du convertisseur boost
  D : Inport
  Add2 : Sum  Inputs=+-
  Constant1 : Constant  Value=1e-6
  Constant2 : Constant
  Controlled Current Source : powerlib/Electrical Sources/Controlled Current Source  Initialize=on  Source_Type=AC  Amplitude=0  Phase=0  Frequency=0  Measurements=None
  Controlled Voltage Source : powerlib/Electrical Sources/Controlled Voltage Source  Initialize=on  Source_Type=AC  Amplitude=0  Phase=0  Frequency=0  Measurements=None
  Current Measurement : powerlib/Measurements/Current Measurement  PhasorSimulation=off  OutputType=Complex  PSBequivalent=0
  Gain : Gain  Gain=0.5
  Iout : UnitDelay  SampleTime=Ts
  Mult : Product  Inputs=**
  Prediction : Subsystem
  Product3 : Product  RndMeth=Zero
  Product5 : Product  Inputs=*/  RndMeth=Zero
  Subtract1 : Sum
  Subtract3 : Sum
  Voltage Measurement : powerlib/Measurements/Voltage Measurement  PhasorSimulation=off  OutputType=Complex  PSBequivalent=0
  Vout : UnitDelay  SampleTime=Ts
  scal : Subsystem
  + : PMIOPort  Tag=PMCPort  Port=1  Side=Right
  - : PMIOPort  Tag=PMCPort  Port=2  Side=Right
  A : PMIOPort  Tag=PMCPort  Port=3  Side=Left
  wires:
  Gain/1 -> Mult/2, Subtract1/2
  Product5/1 -> Iout/1
  Constant1/1 -> Subtract3/2
  Subtract3/1 -> Product5/2
  Product3/1 -> Product5/1  "Pin"
  Prediction/1(Out) -> Subtract3/1
  Vout/1 -> Prediction/1(In), Gain/1
  Subtract1/1 -> Product3/1, Controlled Voltage Source/1  "Vin"
  Mult/1 -> Subtract1/1
  Constant2/1 -> Add2/1
  Add2/1 -> scal/1(D)
  scal/1(m) -> Mult/1
  D/1 -> Add2/2
  Voltage Measurement/1 -> Vout/1
  Iout/1 -> Controlled Current Source/1
  Current Measurement/1 -> Product3/2  "Iin"
  connections:
  -/RConn1 -- Voltage Measurement/LConn2 -- Controlled Voltage Source/LConn1 -- Controlled Current Source/LConn1
  +/RConn1 -- Voltage Measurement/LConn1 -- Controlled Current Source/RConn1
  A/RConn1 -- Current Measurement/LConn1
  Controlled Voltage Source/RConn1 -- Current Measurement/RConn1

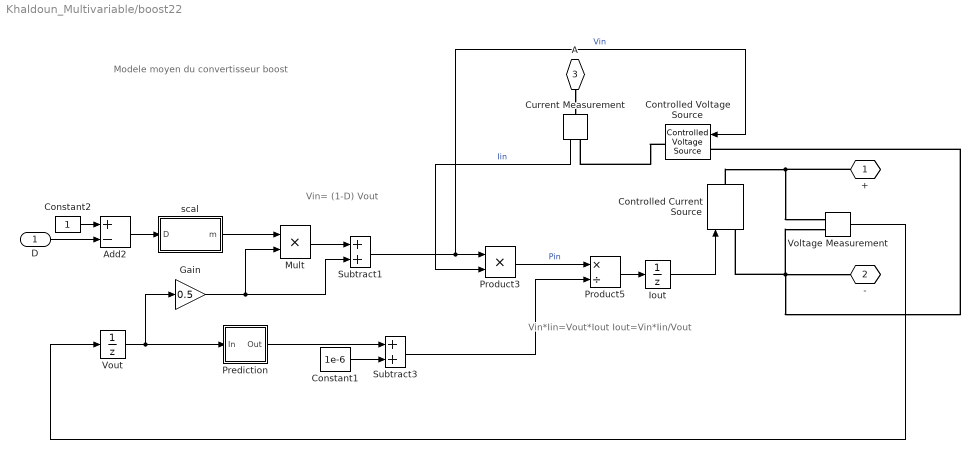
== system Khaldoun_Multivariable/boost22 ==
  note: Modele moyen du convertisseur boost
  note: Vin= (1-D) Vout
  note: Vin*Iin=Vout*Iout
      | Iout=Vin*Iin/Vout
  D : Inport
  Add2 : Sum  Inputs=+-
  Constant1 : Constant  Value=1e-6
  Constant2 : Constant
  Controlled Current Source : powerlib/Electrical Sources/Controlled Current Source  Initialize=on  Source_Type=AC  Amplitude=0  Phase=0  Frequency=0  Measurements=None
  Controlled Voltage Source : powerlib/Electrical Sources/Controlled Voltage Source  Initialize=on  Source_Type=AC  Amplitude=0  Phase=0  Frequency=0  Measurements=None
  Current Measurement : powerlib/Measurements/Current Measurement  PhasorSimulation=off  OutputType=Complex  PSBequivalent=0
  Gain : Gain  Gain=0.5
  Iout : UnitDelay  SampleTime=Ts
  Mult : Product  Inputs=**
  Prediction : Subsystem
  Product3 : Product  RndMeth=Zero
  Product5 : Product  Inputs=*/  RndMeth=Zero
  Subtract1 : Sum
  Subtract3 : Sum
  Voltage Measurement : powerlib/Measurements/Voltage Measurement  PhasorSimulation=off  OutputType=Complex  PSBequivalent=0
  Vout : UnitDelay  SampleTime=Ts
  scal : Subsystem
  + : PMIOPort  Tag=PMCPort  Port=1  Side=Right
  - : PMIOPort  Tag=PMCPort  Port=2  Side=Right
  A : PMIOPort  Tag=PMCPort  Port=3  Side=Left
  wires:
  Current Measurement/1 -> Product3/2  "Iin"
  Iout/1 -> Controlled Current Source/1
  Voltage Measurement/1 -> Vout/1
  D/1 -> Add2/2
  scal/1(m) -> Mult/1
  Add2/1 -> scal/1(D)
  Constant2/1 -> Add2/1
  Mult/1 -> Subtract1/1
  Subtract1/1 -> Controlled Voltage Source/1, Product3/1  "Vin"
  Vout/1 -> Gain/1, Prediction/1(In)
  Prediction/1(Out) -> Subtract3/1
  Product3/1 -> Product5/1  "Pin"
  Subtract3/1 -> Product5/2
  Constant1/1 -> Subtract3/2
  Product5/1 -> Iout/1
  Gain/1 -> Subtract1/2, Mult/2
  connections:
  Controlled Voltage Source/RConn1 -- Current Measurement/RConn1
  A/RConn1 -- Current Measurement/LConn1
  Controlled Current Source/RConn1 -- Voltage Measurement/LConn1 -- +/RConn1
  Controlled Current Source/LConn1 -- Controlled Voltage Source/LConn1 -- Voltage Measurement/LConn2 -- -/RConn1

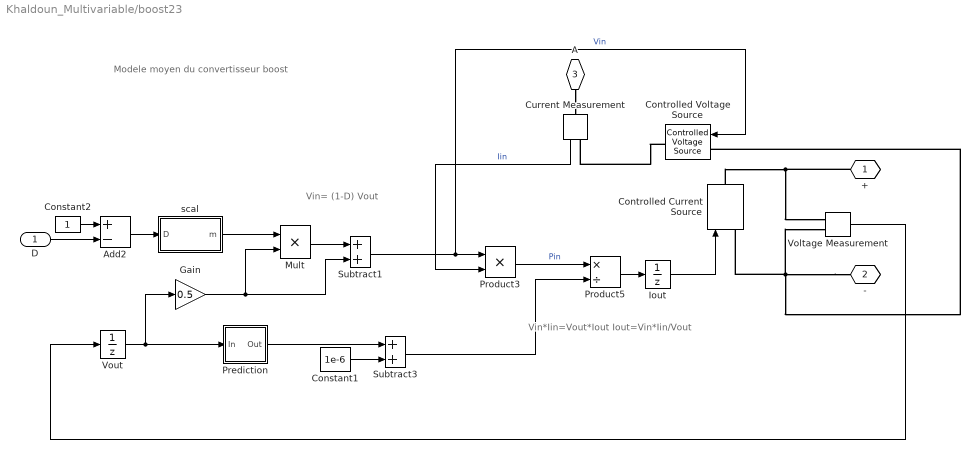
== system Khaldoun_Multivariable/boost23 ==
  note: Vin*Iin=Vout*Iout
      | Iout=Vin*Iin/Vout
  note: Vin= (1-D) Vout
  note: Modele moyen du convertisseur boost
  D : Inport
  Add2 : Sum  Inputs=+-
  Constant1 : Constant  Value=1e-6
  Constant2 : Constant
  Controlled Current Source : powerlib/Electrical Sources/Controlled Current Source  Initialize=on  Source_Type=AC  Amplitude=0  Phase=0  Frequency=0  Measurements=None
  Controlled Voltage Source : powerlib/Electrical Sources/Controlled Voltage Source  Initialize=on  Source_Type=AC  Amplitude=0  Phase=0  Frequency=0  Measurements=None
  Current Measurement : powerlib/Measurements/Current Measurement  PhasorSimulation=off  OutputType=Complex  PSBequivalent=0
  Gain : Gain  Gain=0.5
  Iout : UnitDelay  SampleTime=Ts
  Mult : Product  Inputs=**
  Prediction : Subsystem
  Product3 : Product  RndMeth=Zero
  Product5 : Product  Inputs=*/  RndMeth=Zero
  Subtract1 : Sum
  Subtract3 : Sum
  Voltage Measurement : powerlib/Measurements/Voltage Measurement  PhasorSimulation=off  OutputType=Complex  PSBequivalent=0
  Vout : UnitDelay  SampleTime=Ts
  scal : Subsystem
  + : PMIOPort  Tag=PMCPort  Port=1  Side=Right
  - : PMIOPort  Tag=PMCPort  Port=2  Side=Right
  A : PMIOPort  Tag=PMCPort  Port=3  Side=Left
  wires:
  Gain/1 -> Mult/2, Subtract1/2
  Product5/1 -> Iout/1
  Constant1/1 -> Subtract3/2
  Subtract3/1 -> Product5/2
  Product3/1 -> Product5/1  "Pin"
  Prediction/1(Out) -> Subtract3/1
  Vout/1 -> Prediction/1(In), Gain/1
  Subtract1/1 -> Product3/1, Controlled Voltage Source/1  "Vin"
  Mult/1 -> Subtract1/1
  Constant2/1 -> Add2/1
  Add2/1 -> scal/1(D)
  scal/1(m) -> Mult/1
  D/1 -> Add2/2
  Voltage Measurement/1 -> Vout/1
  Iout/1 -> Controlled Current Source/1
  Current Measurement/1 -> Product3/2  "Iin"
  connections:
  -/RConn1 -- Voltage Measurement/LConn2 -- Controlled Voltage Source/LConn1 -- Controlled Current Source/LConn1
  +/RConn1 -- Voltage Measurement/LConn1 -- Controlled Current Source/RConn1
  A/RConn1 -- Current Measurement/LConn1
  Controlled Voltage Source/RConn1 -- Current Measurement/RConn1

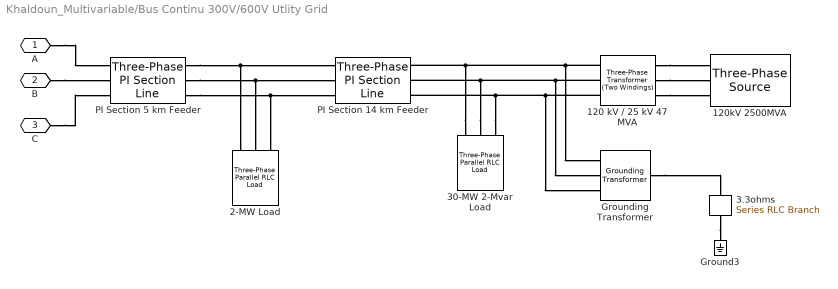
== system Khaldoun_Multivariable/Bus Continu 300V/600V Utlity Grid ==
  120 kV / 25 kV 47 MVA : powerlib/Elements/Three-Phase Transformer (Two Windings)  Winding1Connection=Yg  UNITS=pu  NominalPower=[47e6 60 ]  Winding1="[ 120e3  0.08/30   0.08 ]"  Winding2Connection=Delta (D1)  Winding2="[ 25e3  0.08/30  0.08]"  SetSaturation=off  Rm=500  Lm=500  Saturation="[ 0,0  ;  0.005,1.2  ;  1.0,1.4 ]"  Hysteresis=off  DataFile='basic_model'  SetInitialFlux=off  InitialFluxes=[ 0.8 , -0.8 , 0.7 ]  Measurements=None  MoreParameters=off  BreakLoop=off  DataType=off  TransfoNumber=0
  120kV 2500MVA : powerlib/Electrical Sources/Three-Phase Source  Voltage=120e3  PhaseAngle=0  Frequency=60  InternalConnection=Yg  SpecifyImpedance=on  Resistance=0.8929  Inductance=16.58e-3  ShortCircuitLevel=2500e6  BaseVoltage=120e3  XRratio=7  BusType=swing  Pref=0  Qref=0  Qmin=-inf  Qmax=inf
  2-MW Load : powerlib/Elements/Three-Phase Parallel RLC Load  LConnTagsString=A|B|C  Configuration=Y (grounded)  NominalVoltage=25e3  NominalFrequency=60  ActivePower=2e6  InductivePower=0  CapacitivePower=0  Measurements=None  LoadType=constant Z
  "3.3ohms " : powerlib/Elements/Series RLC Branch  LConnTagsString=__new0  RConnTagsString=__new0  BranchType=R  Resistance=3.3  Inductance=[]  SetiL0=off  InitialCurrent=0  Capacitance=[]  Setx0=off  InitialVoltage=0  Measurements=None
  30-MW 2-Mvar Load : powerlib/Elements/Three-Phase Parallel RLC Load  LConnTagsString=A|B|C  Configuration=Y (grounded)  NominalVoltage=25e3  NominalFrequency=60  ActivePower=30e6  InductivePower=2e6  CapacitivePower=0  Measurements=None  LoadType=constant Z
  Ground3 : powerlib/Elements/Ground  LConnTagsString=a
  "Grounding Transformer " : powerlib/Elements/Grounding Transformer   UNITS=pu  NominalPower="[100e6   60]"  NominalVoltage=25e3  ZeroSequenceImpedance_pu=[0.025 0.75]  MagnetizationBranch_pu=[500 500]  ZeroSequenceImpedance_SI=[0.052083 589.05]  MagnetizationBranch_SI=[1041.7 3.927e+005]  Measurements=None
  PI Section 14 km Feeder : powerlib/Elements/Three-Phase PI Section Line  LConnTagsString=a|b|c  RConnTagsString=A|B|C  Frequency=60  Resistances=[0.1153 0.413]  Inductances=[1.05e-3 3.32e-3]  Capacitances=[11.33e-009 5.01e-009]  Length=14
  PI Section 5 km Feeder : powerlib/Elements/Three-Phase PI Section Line  LConnTagsString=a|b|c  RConnTagsString=A|B|C  Frequency=60  Resistances=[0.1153 0.413]  Inductances=[1.05e-3 3.32e-3]  Capacitances=[11.33e-009 5.01e-009]  Length=5
  A : PMIOPort  Port=1  Side=Left
  B : PMIOPort  Port=2  Side=Left
  C : PMIOPort  Port=3  Side=Left
  connections:
  "Grounding Transformer "/RConn1 -- "3.3ohms "/LConn1
  C/RConn1 -- PI Section 5 km Feeder/LConn3
  B/RConn1 -- PI Section 5 km Feeder/LConn2
  A/RConn1 -- PI Section 5 km Feeder/LConn1
  PI Section 5 km Feeder/RConn3 -- 2-MW Load/LConn3 -- PI Section 14 km Feeder/LConn3
  PI Section 5 km Feeder/RConn2 -- 2-MW Load/LConn2 -- PI Section 14 km Feeder/LConn2
  PI Section 5 km Feeder/RConn1 -- 2-MW Load/LConn1 -- PI Section 14 km Feeder/LConn1
  30-MW 2-Mvar Load/LConn3 -- "Grounding Transformer "/LConn3 -- 120 kV / 25 kV 47 MVA/RConn3 -- PI Section 14 km Feeder/RConn3
  30-MW 2-Mvar Load/LConn2 -- "Grounding Transformer "/LConn2 -- 120 kV / 25 kV 47 MVA/RConn2 -- PI Section 14 km Feeder/RConn2
  30-MW 2-Mvar Load/LConn1 -- "Grounding Transformer "/LConn1 -- 120 kV / 25 kV 47 MVA/RConn1 -- PI Section 14 km Feeder/RConn1
  120 kV / 25 kV 47 MVA/LConn3 -- 120kV 2500MVA/RConn3
  120 kV / 25 kV 47 MVA/LConn2 -- 120kV 2500MVA/RConn2
  120 kV / 25 kV 47 MVA/LConn1 -- 120kV 2500MVA/RConn1
  "3.3ohms "/RConn1 -- Ground3/LConn1

== system Khaldoun_Multivariable/Bus Continu 300V/Boucle de Controle VSC ==
  note: VSC Main Controller
  Vabc_prim : Inport  PortDimensions=3
  Iabc_prim : Inport  Port=2  PortDimensions=3
  Vdc_mes : Inport  Port=3  PortDimensions=1
  Current Regulator : Subsystem
  Iq_ref : Constant  Value=0
  Mux : Mux  Inputs=2
  PLL & Measurements : Subsystem
  Uabc_ref Generation  max (m) = 1 : Subsystem
  Unit Delay : UnitDelay  SampleTime=Ts_Control
  VDC Regulator : Subsystem
  Vdc_ref1 : Constant  Value=Vdc_ref
  Uref : Outport
  wires:
  Vdc_ref1/1 -> VDC Regulator/2(Vdc_ref)
  Uabc_ref Generation  max (m) = 1/1(Uabc_ref) -> Unit Delay/1
  Unit Delay/1 -> Uref/1
  Iabc_prim/1 -> PLL & Measurements/2(Iabc_prim)
  Vabc_prim/1 -> PLL & Measurements/1(Vabc_prim)
  Vdc_mes/1 -> VDC Regulator/1(Vdc_mes)
  PLL & Measurements/2(VdVq_prim) -> Current Regulator/1(VdVq_mes)
  PLL & Measurements/3(IdIq_prim) -> Current Regulator/2(IdIq_mes)
  Mux/1 -> Current Regulator/3(IdIq_ref)
  Iq_ref/1 -> Mux/2
  Current Regulator/1(VdVq_conv) -> Uabc_ref Generation  max (m) = 1/2(VdVq_conv)
  PLL & Measurements/1(wt) -> Uabc_ref Generation  max (m) = 1/1(wt)
  VDC Regulator/1(Id_ref) -> Mux/1

== system Khaldoun_Multivariable/PV1/Diode ==
  note: k = 1.381e-23;      % cste de Boltzmann
      | q = 1.602e-19;      % charge electron
      | A = 1.81;           % facteur de idealité de la diode (1<A<2)
      | Eg = 1.16;          % energie de bandgap du semi-conducteur (eV)
      | Ns = 72;            % cellules en =
      | Np=1;               % cellules en //
      | ki=1.96e-3;         % Coefficient de température de court-circuit(A/°K)
      | Rs =2.48e-3;        % résistance serie(Ohm)
      | Rp = 8.7;           % résistance parallele(Ohm)
      | Tr =298.5;          % temperature de reference en (K)
      | I0_r = 1.13e-6;     % courant inverse de référence
      | Ir_ph = 5.61;       % (A) courant de c-c de référence
      | T = 273 + Tm;       % Temp du module en (K)
  Add : Sum  Inputs=-+
  Id : powerlib/Electrical Sources/Controlled Current Source  Initialize=on  Source_Type=AC  Amplitude=0  Phase=0  Frequency=0  Measurements=None
  Math Function : Math  SaturateOnIntegerOverflow=on
  Product : Product  RndMeth=Zero
  Product1 : Product  Inputs=*/  RndMeth=Zero
  VT : Constant  Value=k*T/q*Ns*A
  Vd : powerlib/Measurements/Voltage Measurement  PhasorSimulation=off  OutputType=Complex  PSBequivalent=0
  courant inv : Constant  Value=I0_r
  one : Constant
  retard : UnitDelay  SampleTime=-1
  A : PMIOPort  Port=1  Side=Left
  K : PMIOPort  Port=2  Side=Right
  wires:
  Product/1 -> Id/1
  Vd/1 -> retard/1
  courant inv/1 -> Product/1  "I0"
  Product1/1 -> Math Function/1
  Add/1 -> Product/2
  VT/1 -> Product1/2
  retard/1 -> Product1/1
  one/1 -> Add/1
  Math Function/1 -> Add/2
  connections:
  K/RConn1 -- Vd/LConn2 -- Id/RConn1
  A/RConn1 -- Id/LConn1 -- Vd/LConn1

== system Khaldoun_Multivariable/PV2/Diode ==
  note: k = 1.381e-23;      % cste de Boltzmann
      | q = 1.602e-19;      % charge electron
      | A = 1.81;           % facteur de idealité de la diode (1<A<2)
      | Eg = 1.16;          % energie de bandgap du semi-conducteur (eV)
      | Ns = 72;            % cellules en =
      | Np=1;               % cellules en //
      | ki=1.96e-3;         % Coefficient de température de court-circuit(A/°K)
      | Rs =2.48e-3;        % résistance serie(Ohm)
      | Rp = 8.7;           % résistance parallele(Ohm)
      | Tr =298.5;          % temperature de reference en (K)
      | I0_r = 1.13e-6;     % courant inverse de référence
      | Ir_ph = 5.61;       % (A) courant de c-c de référence
      | T = 273 + Tm;       % Temp du module en (K)
  Add : Sum  Inputs=-+
  Id : powerlib/Electrical Sources/Controlled Current Source  Initialize=on  Source_Type=AC  Amplitude=0  Phase=0  Frequency=0  Measurements=None
  Math Function : Math  SaturateOnIntegerOverflow=on
  Product : Product  RndMeth=Zero
  Product1 : Product  Inputs=*/  RndMeth=Zero
  VT : Constant  Value=k*T/q*Ns*A
  Vd : powerlib/Measurements/Voltage Measurement  PhasorSimulation=off  OutputType=Complex  PSBequivalent=0
  courant inv : Constant  Value=I0_r
  one : Constant
  retard : UnitDelay  SampleTime=-1
  A : PMIOPort  Port=1  Side=Left
  K : PMIOPort  Port=2  Side=Right
  wires:
  Product/1 -> Id/1
  Vd/1 -> retard/1
  courant inv/1 -> Product/1  "I0"
  Product1/1 -> Math Function/1
  Add/1 -> Product/2
  VT/1 -> Product1/2
  retard/1 -> Product1/1
  one/1 -> Add/1
  Math Function/1 -> Add/2
  connections:
  K/RConn1 -- Vd/LConn2 -- Id/RConn1
  A/RConn1 -- Id/LConn1 -- Vd/LConn1

== system Khaldoun_Multivariable/PV2/Eclairage (W/m2) ==
  Demux : Demux  Tag=STV Demux  Outputs=1
  FromWs : FromWorkspace  Tag=STV FromWs  VariableName=tuvar  SampleTime=0  SigBuilderData=DataTag0  VnvData=DataTag1
      SigBuilderData=|
      | common.afterFinalStr = 'Extrapolate'
      | common.sampleTime = '0'
      | dataSet(1).timeRange = [0 1]
      | dataSet(1).name = 'Constant Irradiance'
      | dataSet(2).timeRange = [0 3]
      | dataSet(2).name = 'Eclairage echelon'
      | sbobj.Groups(1).Name = 'Constant Irradiance'
      | sbobj.Groups(1).Signals.Name = 'Ir'
      | sbobj.Groups(1).Signals.XData = [0 1]
      | sbobj.Groups(1).Signals.YData = [1000 1000]
      | sbobj.Groups(1).TimeRange = [0 1]
      | sbobj.Groups(2).Name = 'Eclairage echelon'
      | sbobj.Groups(2).Signals.Name = 'Ir'
      | sbobj.Groups(2).Signals.XData = [0 0.5 0.5 1 1 1.5 2 2.5 2.7 3]
      | sbobj.Groups(2).Signals.YData = [1 1 0.5 0.5 1 1 1 1 1 1]
      | sbobj.Groups(2).TimeRange = [0 3]
  Ir : Outport  Tag=STV Outport
  wires:
  Demux/1 -> Ir/1
  FromWs/1 -> Demux/1

== system Khaldoun_Multivariable/PV3/Diode ==
  note: k = 1.381e-23;      % cste de Boltzmann
      | q = 1.602e-19;      % charge electron
      | A = 1.81;           % facteur de idealité de la diode (1<A<2)
      | Eg = 1.16;          % energie de bandgap du semi-conducteur (eV)
      | Ns = 72;            % cellules en =
      | Np=1;               % cellules en //
      | ki=1.96e-3;         % Coefficient de température de court-circuit(A/°K)
      | Rs =2.48e-3;        % résistance serie(Ohm)
      | Rp = 8.7;           % résistance parallele(Ohm)
      | Tr =298.5;          % temperature de reference en (K)
      | I0_r = 1.13e-6;     % courant inverse de référence
      | Ir_ph = 5.61;       % (A) courant de c-c de référence
      | T = 273 + Tm;       % Temp du module en (K)
  Add : Sum  Inputs=-+
  Id : powerlib/Electrical Sources/Controlled Current Source  Initialize=on  Source_Type=AC  Amplitude=0  Phase=0  Frequency=0  Measurements=None
  Math Function : Math  SaturateOnIntegerOverflow=on
  Product : Product  RndMeth=Zero
  Product1 : Product  Inputs=*/  RndMeth=Zero
  VT : Constant  Value=k*T/q*Ns*A
  Vd : powerlib/Measurements/Voltage Measurement  PhasorSimulation=off  OutputType=Complex  PSBequivalent=0
  courant inv : Constant  Value=I0_r
  one : Constant
  retard : UnitDelay  SampleTime=-1
  A : PMIOPort  Port=1  Side=Left
  K : PMIOPort  Port=2  Side=Right
  wires:
  Math Function/1 -> Add/2
  one/1 -> Add/1
  retard/1 -> Product1/1
  VT/1 -> Product1/2
  Add/1 -> Product/2
  Product1/1 -> Math Function/1
  courant inv/1 -> Product/1  "I0"
  Vd/1 -> retard/1
  Product/1 -> Id/1
  connections:
  Vd/LConn1 -- Id/LConn1 -- A/RConn1
  Id/RConn1 -- Vd/LConn2 -- K/RConn1

== system Khaldoun_Multivariable/PV4/Diode ==
  note: k = 1.381e-23;      % cste de Boltzmann
      | q = 1.602e-19;      % charge electron
      | A = 1.81;           % facteur de idealité de la diode (1<A<2)
      | Eg = 1.16;          % energie de bandgap du semi-conducteur (eV)
      | Ns = 72;            % cellules en =
      | Np=1;               % cellules en //
      | ki=1.96e-3;         % Coefficient de température de court-circuit(A/°K)
      | Rs =2.48e-3;        % résistance serie(Ohm)
      | Rp = 8.7;           % résistance parallele(Ohm)
      | Tr =298.5;          % temperature de reference en (K)
      | I0_r = 1.13e-6;     % courant inverse de référence
      | Ir_ph = 5.61;       % (A) courant de c-c de référence
      | T = 273 + Tm;       % Temp du module en (K)
  Add : Sum  Inputs=-+
  Id : powerlib/Electrical Sources/Controlled Current Source  Initialize=on  Source_Type=AC  Amplitude=0  Phase=0  Frequency=0  Measurements=None
  Math Function : Math  SaturateOnIntegerOverflow=on
  Product : Product  RndMeth=Zero
  Product1 : Product  Inputs=*/  RndMeth=Zero
  VT : Constant  Value=k*T/q*Ns*A
  Vd : powerlib/Measurements/Voltage Measurement  PhasorSimulation=off  OutputType=Complex  PSBequivalent=0
  courant inv : Constant  Value=I0_r
  one : Constant
  retard : UnitDelay  SampleTime=-1
  A : PMIOPort  Port=1  Side=Left
  K : PMIOPort  Port=2  Side=Right
  wires:
  Product/1 -> Id/1
  Vd/1 -> retard/1
  courant inv/1 -> Product/1  "I0"
  Product1/1 -> Math Function/1
  Add/1 -> Product/2
  VT/1 -> Product1/2
  retard/1 -> Product1/1
  one/1 -> Add/1
  Math Function/1 -> Add/2
  connections:
  K/RConn1 -- Vd/LConn2 -- Id/RConn1
  A/RConn1 -- Id/LConn1 -- Vd/LConn1
